simulink model "Iteration"  (R2018a)
settings: Solver=FixedStepAuto  StartTime=0.0  StopTime=45.0  FixedStep=0.01  RelTol=1e-3
settings Model: Creator=mmyynn  LastModifiedBy=mmyynn

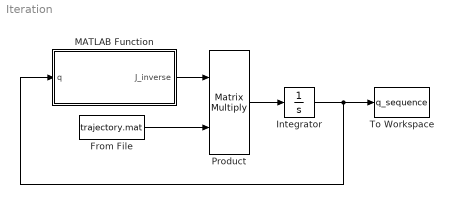
== system Iteration ==
  From File : FromFile  FileName=trajectory.mat  SampleTime=0
  Integrator : Integrator  InitialCondition=[0;pi/2;pi/2;-pi/2;-pi/2;0]
  MATLAB Function : MATLAB Function  TreatAsAtomicUnit=on
  Product : Product  Multiplication=Matrix(*)
  To Workspace : ToWorkspace  VariableName=q_sequence  SampleTime=-1
  wires:
  MATLAB Function/1(J_inverse) -> Product/1
  Product/1 -> Integrator/1
  Integrator/1 -> To Workspace/1, MATLAB Function/1(q)
  From File/1 -> Product/2

== matlab function Iteration/MATLAB Function ==
  data: q input; J_inverse output
function J_inverse=JacobianMatrix(q)
    %DH参数表
    a0=0;       alpha0=0;      d1=0.1807;  
    a1=0;       alpha1=pi/2;   d2=0;       
    a2=0.6126;  alpha2=0;      d3=0;       
    a3=0.5713;  alpha3=0;      d4=0.1741;  
    a4=0;       alpha4=-pi/2;  d5=0.1198;  
    a5=0;       alpha5=pi/2;   d6=0.1165;  
    r=0.22;
%     r=0.195;
%     r=0;
    %
    T01=[cos(q(1)) -sin(q(1)) 0 0;
         sin(q(1)) cos(q(1)) 0 0;
         0 0 1 d1;
         0 0 0 1];
    T12=[cos(q(2)) -sin(q(2)) 0 0;
         0 0 -1 0;
         sin(q(2)) cos(q(2)) 0 0;
         0 0 0 1];
    T23=[cos(q(3)) -sin(q(3)) 0 a2;
         sin(q(3)) cos(q(3)) 0 0;
         0 0 1 0;
         0 0 0 1];
    T3t=[cos(q(4)) -sin(q(4)) 0 a3;
         sin(q(4)) cos(q(4)) 0 0;
         0 0 1 0;
         0 0 0 1];
    Tt4=[1 0 0 0;
         0 1 0 0;
         0 0 1 d4;
         0 0 0 1];
    T45=[cos(q(5)) -sin(q(5)) 0 0;
         0 0 1 d5;
         -sin(q(5)) -cos(q(5)) 0 0;
         0 0 0 1];
    T56=[cos(q(6)) -sin(q(6)) 0 0;
         0 0 -1 -d6;
         sin(q(6)) cos(q(6)) 0 0;
         0 0 0 1];
    T6e=[1 0 0 0;
         0 1 0 0;
         0 0 1 r;
         0 0 0 1];
    T02=T01*T12;
    T03=T02*T23;
    T0t=T03*T3t;
    T04=T0t*Tt4;
    T05=T04*T45;
    T06=T05*T56;
    T0e=T06*T6e;
    
    z1=T01(1:3,3);
    z2=T02(1:3,3);
    z3=T03(1:3,3);
    z4=T04(1:3,3);
    z5=T05(1:3,3);
    z6=T06(1:3,3);
    
    re=T0e(1:3,4);
    
    p1=[0;0;0];
    p2=T01(1:3,4);
    p3=T03(1:3,4);
    p4=T0t(1:3,4);
    p5=T04(1:3,4);
    p6=T05(1:3,4);

    J1=cross(z1,re-p1);
    J2=cross(z2,re-p2);
    J3=cross(z3,re-p3);
    J4=cross(z4,re-p4);
    J5=cross(z5,re-p5);
    J6=cross(z6,re-p6);
    
    JL=[J1 J2 J3 J4 J5 J6];
    JA=[z1 z2 z3 z4 z5 z6];
    J=[JL;JA];
    if(det(J)==0)
        lambda=1e-3;
        J_inverse=J'*inv(J*J'+lambda*eye(6));
    else
        J_inverse=inv(J);
    end
end
